simulink model "OPC_UA_test"  (R2024b)
settings: Solver=FixedStepAuto  StartTime=0.0  StopTime=inf  FixedStep=0.01  RelTol=1e-3
libraries: opcualib x1
settings Model: Creator=student  LastModifiedBy=student

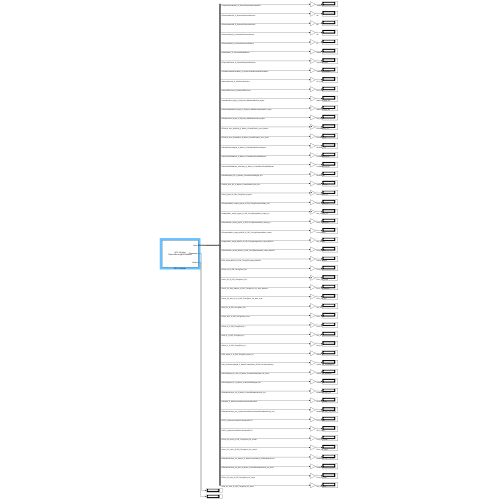
[thumbnail: Simulink's stored preview of the top-level diagram]
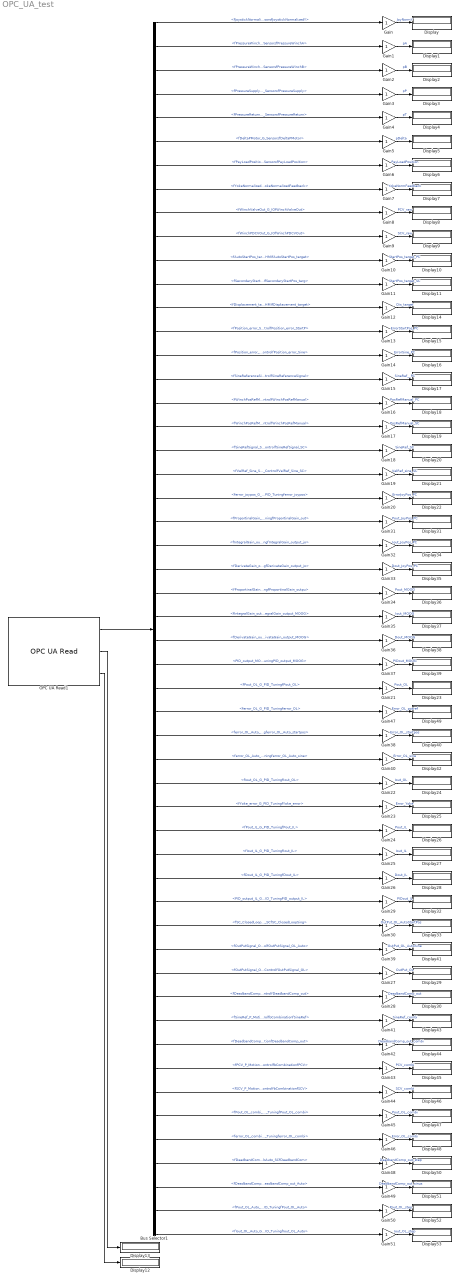
== system OPC_UA_test ==
  Bus Selector1 : BusSelector  OutputSignals=fJoystickNormalizedY_G_SensorsfJoystickNormalizedY,fPressureWinchA_G_SensorsfPressureWinchA,fPressureWinchB_G_SensorsfPressureWinchB,fPressureSupply_G_SensorsfPressureSupply,fPressureReturn_G_SensorsfPressureReturn,fDeltaPMotor_G_SensorsfDeltaPMotor,fPayLoadPosition_G_SensorsfPayLoadPosition,fYokeNormalizedFeedback_G_SensorsfYokeNormalizedFeedback,fWinchValveOut_G_IOfWinchValveOut,fWinchPDCVOut_G_IOfWinchPDCVOut,fAutoStartPos_target_G_Engineer_HMIfAutoStartPos_target,fSecondaryStartPos_target_G_Engineer_HMIfSecondaryStartPos_targ,fDisplacement_target_G_Engineer_HMIfDisplacement_target,fPosition_error_StartPos_G_Motion_ControlfPosition_error_StartP,fPosition_error_SineMotion_G_Motion_ControlfPosition_error_Sine,fSineReferenceSignal_G_Motion_ControlfSineReferenceSignal,fWinchPosRefManual_G_Motion_ControlfWinchPosRefManual,fWinchPosRefManual_secondary_G_Motion_ControlfWinchPosRefManual,fSineRefSignal_SC_G_Motion_ControlfSineRefSignal_SC,fVelRef_Sine_SC_G_Motion_ControlfVelRef_Sine_SC,ferror_joypos_G_PID_Tuningferror_joypos,fProportinalGain_output_joypos_G_PID_TuningfProportinalGain_out,fIntegralGain_output_joypos_G_PID_TuningfIntegralGain_output_jo,fDerivateGain_output_joypos_G_PID_TuningfDerivateGain_output_jo,fProportinalGain_output_MOOG_G_PID_TuningfProportinalGain_outpu,fIntegralGain_output_MOOG_G_PID_TuningfIntegralGain_output_MOOG,fDerivateGain_output_MOOG_G_PID_TuningfDerivateGain_output_MOOG,PID_output_MOOG_G_PID_TuningPID_output_MOOG,fPout_OL_G_PID_TuningfPout_OL,ferror_OL_G_PID_Tuningferror_OL,ferror_OL_Auto_startpos_G_PID_Tuningferror_OL_Auto_startpos,ferror_OL_Auto_sine_G_PID_Tuningferror_OL_Auto_sine,fIout_OL_G_PID_TuningfIout_OL,fYoke_error_G_PID_TuningfYoke_error,fPout_IL_G_PID_TuningfPout_IL,fIout_IL_G_PID_TuningfIout_IL,fDout_IL_G_PID_TuningfDout_IL,PID_output_IL_G_PID_TuningPID_output_IL,fSC_ClosedLoopSingal_P_MotionControlfbAuto_SCfSC_ClosedLoopSing,fOutPutSignal_OL_Auto_G_Motion_ControlfOutPutSignal_OL_Auto,fOutPutSignal_OL_G_Motion_ControlfOutPutSignal_OL,fDeadbandComp_out_G_Motion_ControlfDeadbandComp_out,fSineRef_P_MotionControlfbCombinationfSineRef,fDeadbandComp_out_P_MotionControlfbCombinationfDeadbandComp_out,fPCV_P_MotionControlfbCombinationfPCV,fSCV_P_MotionControlfbCombinationfSCV,fPout_OL_combi_G_PID_TuningfPout_OL_combi,ferror_OL_combi_G_PID_Tuningferror_OL_combi,fDeadbandComp_out_startpos_P_MotionControlfbAuto_SCfDeadbandCom,fDeadbandComp_out_Auto_G_Motion_ControlfDeadbandComp_out_Auto,fPout_OL_Auto_G_PID_TuningfPout_OL_Auto,fIout_OL_Auto_G_PID_TuningfIout_OL_Auto
  Display{,1..53} (54 alike) : Display
  Gain{,1..51} (52 alike) : Gain
  OPC UA Read1 : opcualib/OPC UA Read  SelectedServer=TcOpcUaServer@CX5240MRH  ServerList=TcOpcUaServer@CX5240MRH  NodeList={ '1', 'fJoystickNormalizedY', '4', 'G_Sensors.fJoystickNormalizedY', '0'; '2', 'fPressureWinchA', '4', 'G_Sensors.fPressureWinchA', '0'; '3', 'fPressureWinchB', '4', 'G_Sensors.fPressureWinchB', '0'; '4', 'fPressureSupply', '4', 'G_Sensors.fPressureSupply', '0'; '5', 'fPressureReturn', '4', 'G_Sensors.fPressureReturn', '0'; '6', 'fDeltaPMotor', '4', 'G_Sensors.fDeltaPMotor', '0'; '7', 'fPayLoadPosition', '4', 'G_Sensors.fPayLoadPosition', '0'; '8', 'fYokeNormalizedFeedback', '4', 'G_Sensors.fYokeNormalizedFeedback', '0'; '9', 'fWinchValveOut', '4', 'G_IO.fWinchValveOut', '0'; '10', 'fWinchPDCVOut', '4', 'G_IO.fWinchPDCVOut', '0'; '11', 'fAutoStartPos_target', '4', 'G_Engineer_HMI.fAutoStartPos_target', '0'; '12', 'fSecondaryStartPos_target', '4', 'G_Engineer_HMI.fSecondaryStartPos_target', '0'; '13', 'fDisplacement_target', '4', 'G_Engineer_HMI.fDisplacement_target', '0'; '14', 'fPosition_error_StartPos', '4', 'G_Motion_Control.fPosition_error_StartPos', '0'; '15', 'fPosition_error_SineMotion', '4', 'G_Motion_Control.fPosition_error_SineMotion', '0'; '16', 'fSineReferenceSignal', '4', 'G_Motion_Control.fSineReferenceSignal', '0'; '17', 'fWinchPosRefManual', '4', 'G_Motion_Control.fWinchPosRefManual', '0'; '18', 'fWinchPosRefManual_secondary', '4', 'G_Motion_Control.fWinchPosRefManual_secondary', '0'; '19', 'fSineRefSignal_SC', '4', 'G_Motion_Control.fSineRefSignal_SC', '0'; '20', 'fVelRef_Sine_SC', '4', 'G_Motion_Control.fVelRef_Sine_SC', '0'; '21', 'ferror_joypos', '4', 'G_PID_Tuning.ferror_joypos', '0'; '22', 'fProportinalGain_output_joypos', '4', 'G_PID_Tuning.fProportinalGain_output_joypos', '0'; '23', 'fIntegralGain_output_joypos', '4', 'G_PID_Tuning.fIntegralGain_output_joypos', '0'; '24', 'fDerivateGain_output_joypos', '4', 'G_PID_Tuning.fDerivateGain_output_joypos', '0'; '25', 'fProportinalGain_output_MOOG', '4', 'G_PID_Tuning.fProportinalGain_output_MOOG', '0'; '26', 'fIntegralGain_output_MOOG', '4', 'G_PID_Tuning.fIntegralGain_output_MOOG', '0'; '27', 'fDerivateGain_output_MOOG', '4', 'G_PID_Tuning.fDerivateGain_output_MOOG', '0'; '28', 'PID_output_MOOG', '4', 'G_PID_Tuning.PID_output_MOOG', '0'; '29', 'fPout_OL', '4', 'G_PID_Tuning.fPout_OL', '0'; '30', 'fIout_OL', '4', 'G_PID_Tuning.fIout_OL', '0'; '31', 'fYoke_error', '4', 'G_PID_Tuning.fYoke_error', '0'; '32', 'fPout_IL', '4', 'G_PID_Tuning.fPout_IL', '0'; '33', 'fIout_IL', '4', 'G_PID_Tuning.fIout_IL', '0'; '34', 'fDout_IL', '4', 'G_PID_Tuning.fDout_IL', '0'; '35', 'fOutPutSignal_OL', '4', 'G_Motion_Control.fOutPutSignal_OL', '0'; '36', 'fDeadbandComp_out', '4', 'G_Motion_Control.fDeadbandComp_out', '0'; '37', 'PID_output_IL', '4', 'G_PID_Tuning.PID_output_IL', '0'; '38', 'fSC_ClosedLoopSingal', '4', 'P_MotionControl.fbAuto_SC.fSC_ClosedLoopSingal', '0'; '39', 'fOutPutSignal_OL_Auto', '4', 'G_Motion_Control.fOutPutSignal_OL_Auto', '0'; '40', 'ferror_OL_Auto_startpos', '4', 'G_PID_Tuning.ferror_OL_Auto_startpos', '0'; '41', 'ferror_OL_Auto_sine', '4', 'G_PID_Tuning.ferror_OL_Auto_sine', '0'; '42', 'fSineRef', '4', 'P_MotionControl.fbCombination.fSineRef', '0'; '43', 'fDeadbandComp_out', '4', 'P_MotionControl.fbCombination.fDeadbandComp_out', '0'; '44', 'fPCV', '4', 'P_MotionControl.fbCombination.fPCV', '0'; '45', 'fSCV', '4', 'P_MotionControl.fbCombination.fSCV', '0'; '46', 'fPout_OL_combi', '4', 'G_PID_Tuning.fPout_OL_combi', '0'; '47', 'ferror_OL_combi', '4', 'G_PID_Tuning.ferror_OL_combi', '0'; '48', 'ferror_OL', '4', 'G_PID_Tuning.ferror_OL', '0'; '49', 'fDeadbandComp_out_startpos', '4', 'P_MotionControl.fbAuto_SC.fDeadbandComp_out_startpos', '0'; '50', 'fDeadbandComp_out_Auto', '4', 'G_Motion_Control.fDeadbandComp_out_Auto', '0'; '51', 'fPout_OL_Auto', '4', 'G_PID_Tuning.fPout_OL_Auto', '0'; '52', 'fIout_OL_Auto', '4', 'G_PID_Tuning.fIout_OL_Auto', '0' }  ShowQualityPort=on  ShowTimestampPort=on  ShowTimestampPortAs=Seconds since start  SampleTime=-1
  wires:
  Gain5/1 -> Display5/1  "pDelta"
  OPC UA Read1/3 -> Display12/1
  Bus Selector1/44 -> Gain42/1  "<fDeadbandComp_out_P_MotionControlfbCombinationfDeadbandComp_out>"
  Bus Selector1/42 -> Gain28/1  "<fDeadbandComp_out_G_Motion_ControlfDeadbandComp_out>"
  Bus Selector1/40 -> Gain39/1  "<fOutPutSignal_OL_Auto_G_Motion_ControlfOutPutSignal_OL_Auto>"
  Bus Selector1/38 -> Gain29/1  "<PID_output_IL_G_PID_TuningPID_output_IL>"
  OPC UA Read1/2 -> Display13/1
  Gain49/1 -> Display51/1  "DeadbandComp_out_sinus"
  Gain7/1 -> Display7/1  "YokeNormFeedback"
  Bus Selector1/2 -> Gain1/1  "<fPressureWinchA_G_SensorsfPressureWinchA>"
  Bus Selector1/4 -> Gain3/1  "<fPressureSupply_G_SensorsfPressureSupply>"
  Gain1/1 -> Display1/1  "pA"
  Bus Selector1/1 -> Gain/1  "<fJoystickNormalizedY_G_SensorsfJoystickNormalizedY>"
  Bus Selector1/3 -> Gain2/1  "<fPressureWinchB_G_SensorsfPressureWinchB>"
  Gain20/1 -> Display22/1  "ErrorJoyPos_PC"
  Bus Selector1/11 -> Gain10/1  "<fAutoStartPos_target_G_Engineer_HMIfAutoStartPos_target>"
  Bus Selector1/9 -> Gain8/1  "<fWinchValveOut_G_IOfWinchValveOut>"
  Bus Selector1/7 -> Gain6/1  "<fPayLoadPosition_G_SensorsfPayLoadPosition>"
  Bus Selector1/5 -> Gain4/1  "<fPressureReturn_G_SensorsfPressureReturn>"
  Bus Selector1/12 -> Gain11/1  "<fSecondaryStartPos_target_G_Engineer_HMIfSecondaryStartPos_targ>"
  Bus Selector1/10 -> Gain9/1  "<fWinchPDCVOut_G_IOfWinchPDCVOut>"
  Bus Selector1/8 -> Gain7/1  "<fYokeNormalizedFeedback_G_SensorsfYokeNormalizedFeedback>"
  Bus Selector1/6 -> Gain5/1  "<fDeltaPMotor_G_SensorsfDeltaPMotor>"
  Bus Selector1/19 -> Gain18/1  "<fSineRefSignal_SC_G_Motion_ControlfSineRefSignal_SC>"
  Gain17/1 -> Display19/1  "PosRefManual_SC"
  Bus Selector1/17 -> Gain16/1  "<fWinchPosRefManual_G_Motion_ControlfWinchPosRefManual>"
  Bus Selector1/15 -> Gain14/1  "<fPosition_error_SineMotion_G_Motion_ControlfPosition_error_Sine>"
  Bus Selector1/13 -> Gain12/1  "<fDisplacement_target_G_Engineer_HMIfDisplacement_target>"
  Bus Selector1/20 -> Gain19/1  "<fVelRef_Sine_SC_G_Motion_ControlfVelRef_Sine_SC>"
  Gain15/1 -> Display17/1  "SineRef__PC"
  Bus Selector1/18 -> Gain17/1  "<fWinchPosRefManual_secondary_G_Motion_ControlfWinchPosRefManual>"
  Bus Selector1/16 -> Gain15/1  "<fSineReferenceSignal_G_Motion_ControlfSineReferenceSignal>"
  Bus Selector1/14 -> Gain13/1  "<fPosition_error_StartPos_G_Motion_ControlfPosition_error_StartP>"
  Bus Selector1/27 -> Gain36/1  "<fDerivateGain_output_MOOG_G_PID_TuningfDerivateGain_output_MOOG>"
  Gain31/1 -> Display31/1  "Pout_JoyPos_PC"
  Bus Selector1/25 -> Gain34/1  "<fProportinalGain_output_MOOG_G_PID_TuningfProportinalGain_outpu>"
  Bus Selector1/23 -> Gain32/1  "<fIntegralGain_output_joypos_G_PID_TuningfIntegralGain_output_jo>"
  Bus Selector1/21 -> Gain20/1  "<ferror_joypos_G_PID_Tuningferror_joypos>"
  Bus Selector1/26 -> Gain35/1  "<fIntegralGain_output_MOOG_G_PID_TuningfIntegralGain_output_MOOG>"
  Gain3/1 -> Display3/1  "pP"
  Bus Selector1/28 -> Gain37/1  "<PID_output_MOOG_G_PID_TuningPID_output_MOOG>"
  Bus Selector1/24 -> Gain33/1  "<fDerivateGain_output_joypos_G_PID_TuningfDerivateGain_output_jo>"
  Bus Selector1/22 -> Gain31/1  "<fProportinalGain_output_joypos_G_PID_TuningfProportinalGain_out>"
  Bus Selector1/35 -> Gain24/1  "<fPout_IL_G_PID_TuningfPout_IL>"
  Bus Selector1/33 -> Gain22/1  "<fIout_OL_G_PID_TuningfIout_OL>"
  Bus Selector1/31 -> Gain38/1  "<ferror_OL_Auto_startpos_G_PID_Tuningferror_OL_Auto_startpos>"
  Bus Selector1/29 -> Gain21/1  "<fPout_OL_G_PID_TuningfPout_OL>"
  Bus Selector1/36 -> Gain25/1  "<fIout_IL_G_PID_TuningfIout_IL>"
  Bus Selector1/34 -> Gain23/1  "<fYoke_error_G_PID_TuningfYoke_error>"
  Bus Selector1/32 -> Gain40/1  "<ferror_OL_Auto_sine_G_PID_Tuningferror_OL_Auto_sine>"
  Bus Selector1/30 -> Gain47/1  "<ferror_OL_G_PID_Tuningferror_OL>"
  Bus Selector1/41 -> Gain27/1  "<fOutPutSignal_OL_G_Motion_ControlfOutPutSignal_OL>"
  Gain6/1 -> Display6/1  "PayLoadPosition"
  Bus Selector1/43 -> Gain41/1  "<fSineRef_P_MotionControlfbCombinationfSineRef>"
  Bus Selector1/39 -> Gain30/1  "<fSC_ClosedLoopSingal_P_MotionControlfbAuto_SCfSC_ClosedLoopSing>"
  Bus Selector1/37 -> Gain26/1  "<fDout_IL_G_PID_TuningfDout_IL>"
  Bus Selector1/47 -> Gain45/1  "<fPout_OL_combi_G_PID_TuningfPout_OL_combi>"
  Bus Selector1/45 -> Gain43/1  "<fPCV_P_MotionControlfbCombinationfPCV>"
  Bus Selector1/48 -> Gain46/1  "<ferror_OL_combi_G_PID_Tuningferror_OL_combi>"
  Bus Selector1/46 -> Gain44/1  "<fSCV_P_MotionControlfbCombinationfSCV>"
  Bus Selector1/49 -> Gain48/1  "<fDeadbandComp_out_startpos_P_MotionControlfbAuto_SCfDeadbandCom>"
  Bus Selector1/50 -> Gain49/1  "<fDeadbandComp_out_Auto_G_Motion_ControlfDeadbandComp_out_Auto>"
  Gain/1 -> Display/1  "JoyNormY"
  Gain2/1 -> Display2/1  "pB"
  Gain4/1 -> Display4/1  "pT"
  Gain8/1 -> Display8/1  "PCV_raw"
  Gain9/1 -> Display9/1  "SCV_raw"
  Gain10/1 -> Display10/1  "StartPos_target_PC"
  Gain11/1 -> Display11/1  "StartPos_target_SC"
  Gain12/1 -> Display14/1  "Dis_target"
  Gain13/1 -> Display15/1  "ErrorStartPos_PC"
  Gain14/1 -> Display16/1  "ErrorSine_PC"
  Gain16/1 -> Display18/1  "PosRefManual_PC"
  Gain18/1 -> Display20/1  "SineRef_SC"
  Gain19/1 -> Display21/1  "VelRef_sine_SC"
  Gain32/1 -> Display34/1  "Iout_JoyPos_PC"
  Gain33/1 -> Display35/1  "Dout_JoyPos_PC"
  Gain34/1 -> Display36/1  "Pout_MOOG"
  Gain35/1 -> Display37/1  "Iout_MOOG"
  Gain36/1 -> Display38/1  "Dout_MOOG"
  Gain37/1 -> Display39/1  "PIDout_MOOG"
  Gain21/1 -> Display23/1  "Pout_OL"
  Gain47/1 -> Display49/1  "Error_OL_posref"
  Gain38/1 -> Display40/1  "Error_OL_startpos"
  Gain40/1 -> Display42/1  "Error_OL_sine"
  Gain22/1 -> Display24/1  "Iout_OL"
  Gain23/1 -> Display25/1  "Error_Yoke"
  Gain24/1 -> Display26/1  "Pout_IL"
  Gain25/1 -> Display27/1  "Iout_IL"
  Gain26/1 -> Display28/1  "Dout_IL"
  Gain29/1 -> Display32/1  "PIDout_IL"
  Gain30/1 -> Display33/1  "OutPut_OL_AutoStartPos"
  Gain39/1 -> Display41/1  "OutPut_OL_AutoSine"
  Gain27/1 -> Display29/1  "OutPut_OL"
  Gain28/1 -> Display30/1  "DeadbandComp_out"
  Gain41/1 -> Display43/1  "SineRef_combi"
  Gain42/1 -> Display44/1  "DeadbandComp_out_combi"
  Gain43/1 -> Display45/1  "PCV_combi"
  Gain44/1 -> Display46/1  "SCV_combi"
  Gain45/1 -> Display47/1  "Pout_OL_combi"
  Gain46/1 -> Display48/1  "Error_OL_combi"
  Gain48/1 -> Display50/1  "DeadbandComp_out_step"
  Gain50/1 -> Display52/1  "Pout_OL_step"
  Gain51/1 -> Display53/1  "Iout_OL_step"
  Bus Selector1/51 -> Gain50/1  "<fPout_OL_Auto_G_PID_TuningfPout_OL_Auto>"
  Bus Selector1/52 -> Gain51/1  "<fIout_OL_Auto_G_PID_TuningfIout_OL_Auto>"
  OPC UA Read1/1 -> Bus Selector1/1
